simulink model "Simulador_MotorDC_Equivalent_BLDC"  (R2019a)
settings: Solver=VariableStepAuto  StartTime=0.0  StopTime=100  RelTol=1e-3
values from neighbouring files (symbols this model uses):
  b = 3.2*10^(-3)    (= 0.0032)    [Simulador_MotorDC_Equivalent_BLDC.m]
  B_fault = 0    [Simulador_MotorDC_Equivalent_BLDC.m]
  B_nonlinear = 1    [Simulador_MotorDC_Equivalent_BLDC.m]
  delta_load = 0.05    [Simulador_MotorDC_Equivalent_BLDC.m]
  f_i = 0    [Simulador_MotorDC_Equivalent_BLDC.m]
  J = 50*10^(-3)*10^(-4)    (= 5e-06)    [Simulador_MotorDC_Equivalent_BLDC.m]
  J_fault = 0    [Simulador_MotorDC_Equivalent_BLDC.m]
  J_nonlinear = 1    [Simulador_MotorDC_Equivalent_BLDC.m]
  Ke = 0.0745    [Simulador_MotorDC_Equivalent_BLDC.m]
  Kt = 74.5*10^(-3)    (= 0.0745)    [Simulador_MotorDC_Equivalent_BLDC.m]
  L = length(r1)    [Algorisme_FDI.m]    (also in Simulador_MotorDC_Equivalent_BLDC.m = 0.0076)
  L_fault = 0    [Simulador_MotorDC_Equivalent_BLDC.m]
  L_nonlinear = 1    [Simulador_MotorDC_Equivalent_BLDC.m]
  Load_fault = 2*delta_load    (= 0.1)    [Simulador_MotorDC_Equivalent_BLDC.m]
  noise_amp = 0.07    [Simulador_MotorDC_Equivalent_BLDC.m]
  P_V_encoder = 1024    [Simulador_MotorDC_Equivalent_BLDC.m]
  pos_stuck = 0    [Simulador_MotorDC_Equivalent_BLDC.m]
  R = 2*1.72    (= 3.44)    [Simulador_MotorDC_Equivalent_BLDC.m]
  R_fault = 0    [Simulador_MotorDC_Equivalent_BLDC.m]
  R_nonlinear = 1    [Simulador_MotorDC_Equivalent_BLDC.m]
  ramp_f_B = 0    [Simulador_MotorDC_Equivalent_BLDC.m]
  ramp_f_J = 0    [Simulador_MotorDC_Equivalent_BLDC.m]
  ramp_f_L = 0    [Simulador_MotorDC_Equivalent_BLDC.m]
  ramp_f_Load = abrup_incip    (= 1)    [Simulador_MotorDC_Equivalent_BLDC.m]
  ramp_f_R = 0    [Simulador_MotorDC_Equivalent_BLDC.m]
  ramp_f_Vdc = 0    [Simulador_MotorDC_Equivalent_BLDC.m]
  ramp_i = 0    [Simulador_MotorDC_Equivalent_BLDC.m]
  stuck_duration = 1    [Simulador_MotorDC_Equivalent_BLDC.m]
  t_fault = 10    [Simulador_MotorDC_Equivalent_BLDC.m]
  tol_B = 0.05    [Simulador_MotorDC_Equivalent_BLDC.m]
  tol_J = 0.05    [Simulador_MotorDC_Equivalent_BLDC.m]
  tol_L = 0.05    [Simulador_MotorDC_Equivalent_BLDC.m]
  tol_R = 0.01    [Simulador_MotorDC_Equivalent_BLDC.m]
  Tsc = 0.0001    [Simulador_MotorDC_Equivalent_BLDC.m]
  Tsd = 0.0001    [Algorisme_FDI.m]    (also in Simulador_MotorDC_Equivalent_BLDC.m)
  Vdc_fault = 0    [Simulador_MotorDC_Equivalent_BLDC.m]
  vel_B = 0.001    [Simulador_MotorDC_Equivalent_BLDC.m]
  vel_i = 0    [Simulador_MotorDC_Equivalent_BLDC.m]
  vel_J = 0.5    [Simulador_MotorDC_Equivalent_BLDC.m]
  vel_L = 0.1    [Simulador_MotorDC_Equivalent_BLDC.m]
  vel_Load = 0.1    [Simulador_MotorDC_Equivalent_BLDC.m]
  vel_R = 0.001    [Simulador_MotorDC_Equivalent_BLDC.m]
  vel_Vdc = 0.001    [Simulador_MotorDC_Equivalent_BLDC.m]
libraries: simulink x2
settings Model: Creator=quimb  LastModifiedBy=Usuario

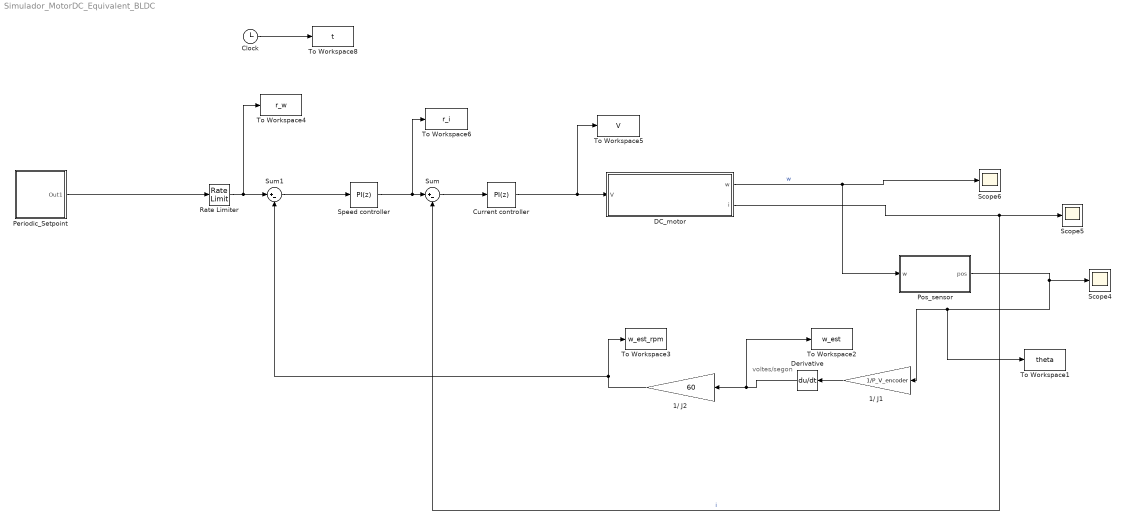
== system Simulador_MotorDC_Equivalent_BLDC ==
  note: voltes/segon
  1/ J1 : Gain  Gain=1/P_V_encoder
  1/ J2 : Gain  Gain=60
  Clock : Clock
  Current controller : simulink/Continuous/PID Controller  Controller=PI  Form=Parallel  TimeDomain=Discrete-time  SampleTime=Tsc  IntegratorMethod=Forward Euler  FilterMethod=Forward Euler  ControllerParametersSource=internal  P=0.1  I=0.1  D=0.5  UseFilter=on  N=100  TunerSelectOption=Transfer Function Based (PID Tuner App)  InitialConditionSource=internal  InitialConditionForIntegrator=0  InitialConditionForFilter=0  DifferentiatorICPrevScaledInput=0  ExternalReset=none  TrackingMode=off  Kt=1  LimitOutput=on  UpperSaturationLimit=24  LowerSaturationLimit=-24  LinearizeAsGain=on  AntiWindupMode=back-calculation  Kb=100  POutMin=[]  POutMax=[]  IOutMin=[]  IOutMax=[]  DOutMin=[]  DOutMax=[]  NOutMin=[]  NOutMax=[]  SumOutMin=[]  SumOutMax=[]  SaturationOutMin=[]  SaturationOutMax=[]  PParamMin=[]  PParamMax=[]  IParamMin=[]  IParamMax=[]  DParamMin=[]  DParamMax=[]  NParamMin=[]  NParamMax=[]  KbParamMin=[]  KbParamMax=[]  KtParamMin=[]  KtParamMax=[]  KbOutMin=[]  KbOutMax=[]  KtOutMin=[]  KtOutMax=[]  IntegratorOutMin=[]  IntegratorOutMax=[]  FilterOutMin=[]  FilterOutMax=[]  SumI1OutMin=[]  SumI1OutMax=[]  SumI2OutMin=[]  SumI2OutMax=[]  SumI3OutMin=[]  SumI3OutMax=[]  SumI4OutMin=[]  SumI4OutMax=[]  SumDOutMin=[]  SumDOutMax=[]  DifferentiatorOutMin=[]  DifferentiatorOutMax=[]  FilterDiffOutCoefMin=[]  FilterDiffOutCoefMax=[]  ReciprocalOutMin=[]  ReciprocalOutMax=[]  SumDenOutMin=[]  SumDenOutMax=[]  SumNumOutMin=[]  SumNumOutMax=[]  DivideOutMin=[]  DivideOutMax=[]  IntegratorContinuousStateAttributes=''  IntegratorStateMustResolveToSignalObject=off  IntegratorRTWStateStorageClass=Auto  FilterContinuousStateAttributes=''  FilterStateMustResolveToSignalObject=off  FilterRTWStateStorageClass=Auto  ParallelPVariant=InternalParameters  IdealPVariant=Disabled  IVariant=InternalParameters  DVariant=Disabled  IntegratorVariant=Discrete  SatVariant=Enabled  AWVariant=BackCalculation  PCopyVariant=Disabled  TRVariant=Disabled  FdbkBlocksVariant=Forward  IdealPFdbkVariant=Disabled  SatFdbkVariant=Disabled  DerivativeFilterVariant=Disabled  NVariant=Disabled  NCopyVariant=Disabled_SignalSpec  FilterICVariant=Disabled  IntegratorICVariant=InternalICs  ExternalResetVariant=Disabled  TRSumVariant=Passthrough  SumFdbkVariant=Disabled  SumVariant=Sum_PI
  DC_motor : Subsystem
  Derivative : Derivative
  Periodic_Setpoint : Subsystem
  Pos_sensor : Subsystem
  Rate Limiter : RateLimiter  RisingSlewLimit=500  FallingSlewLimit=-500  SampleTimeMode=inherited
  Scope4 : Scope
  Scope5 : Scope
  Scope6 : Scope
  Speed controller : simulink/Continuous/PID Controller  Controller=PI  Form=Parallel  TimeDomain=Discrete-time  SampleTime=Tsc  IntegratorMethod=Forward Euler  FilterMethod=Forward Euler  ControllerParametersSource=internal  P=0.5  I=2  D=0.5  UseFilter=on  N=100  TunerSelectOption=Transfer Function Based (PID Tuner App)  InitialConditionSource=internal  InitialConditionForIntegrator=0  InitialConditionForFilter=0  DifferentiatorICPrevScaledInput=0  ExternalReset=none  TrackingMode=off  Kt=1  LimitOutput=on  UpperSaturationLimit=100  LowerSaturationLimit=-100  LinearizeAsGain=on  AntiWindupMode=back-calculation  Kb=100  POutMin=[]  POutMax=[]  IOutMin=[]  IOutMax=[]  DOutMin=[]  DOutMax=[]  NOutMin=[]  NOutMax=[]  SumOutMin=[]  SumOutMax=[]  SaturationOutMin=[]  SaturationOutMax=[]  PParamMin=[]  PParamMax=[]  IParamMin=[]  IParamMax=[]  DParamMin=[]  DParamMax=[]  NParamMin=[]  NParamMax=[]  KbParamMin=[]  KbParamMax=[]  KtParamMin=[]  KtParamMax=[]  KbOutMin=[]  KbOutMax=[]  KtOutMin=[]  KtOutMax=[]  IntegratorOutMin=[]  IntegratorOutMax=[]  FilterOutMin=[]  FilterOutMax=[]  SumI1OutMin=[]  SumI1OutMax=[]  SumI2OutMin=[]  SumI2OutMax=[]  SumI3OutMin=[]  SumI3OutMax=[]  SumI4OutMin=[]  SumI4OutMax=[]  SumDOutMin=[]  SumDOutMax=[]  DifferentiatorOutMin=[]  DifferentiatorOutMax=[]  FilterDiffOutCoefMin=[]  FilterDiffOutCoefMax=[]  ReciprocalOutMin=[]  ReciprocalOutMax=[]  SumDenOutMin=[]  SumDenOutMax=[]  SumNumOutMin=[]  SumNumOutMax=[]  DivideOutMin=[]  DivideOutMax=[]  IntegratorContinuousStateAttributes=''  IntegratorStateMustResolveToSignalObject=off  IntegratorRTWStateStorageClass=Auto  FilterContinuousStateAttributes=''  FilterStateMustResolveToSignalObject=off  FilterRTWStateStorageClass=Auto  ParallelPVariant=InternalParameters  IdealPVariant=Disabled  IVariant=InternalParameters  DVariant=Disabled  IntegratorVariant=Discrete  SatVariant=Enabled  AWVariant=BackCalculation  PCopyVariant=Disabled  TRVariant=Disabled  FdbkBlocksVariant=Forward  IdealPFdbkVariant=Disabled  SatFdbkVariant=Disabled  DerivativeFilterVariant=Disabled  NVariant=Disabled  NCopyVariant=Disabled_SignalSpec  FilterICVariant=Disabled  IntegratorICVariant=InternalICs  ExternalResetVariant=Disabled  TRSumVariant=Passthrough  SumFdbkVariant=Disabled  SumVariant=Sum_PI
  Sum : Sum  Inputs=|+-
  Sum1 : Sum  Inputs=|+-
  To Workspace1 : ToWorkspace  VariableName=theta  SampleTime=Tsd
  To Workspace2 : ToWorkspace  VariableName=w_est  SampleTime=Tsd
  To Workspace3 : ToWorkspace  VariableName=w_est_rpm  SampleTime=Tsd
  To Workspace4 : ToWorkspace  VariableName=r_w  SampleTime=Tsd
  To Workspace5 : ToWorkspace  VariableName=V  SampleTime=Tsd
  To Workspace6 : ToWorkspace  VariableName=r_i  SampleTime=Tsd
  To Workspace8 : ToWorkspace  VariableName=t  SampleTime=Tsd
  wires:
  DC_motor/1(w) -> Pos_sensor/1("w "), Scope6/1  "w"
  Clock/1 -> To Workspace8/1
  1/ J1/1 -> Derivative/1
  Pos_sensor/1(pos) -> To Workspace1/1, 1/ J1/1, Scope4/1
  Derivative/1 -> To Workspace2/1, 1/ J2/1
  1/ J2/1 -> Sum1/2, To Workspace3/1
  DC_motor/2(i) -> Scope5/1, Sum/2  "i"
  Current controller/1 -> To Workspace5/1, DC_motor/1(V)
  Sum1/1 -> Speed controller/1
  Periodic_Setpoint/1(Out1) -> Rate Limiter/1
  Rate Limiter/1 -> To Workspace4/1, Sum1/1
  Speed controller/1 -> To Workspace6/1, Sum/1
  Sum/1 -> Current controller/1

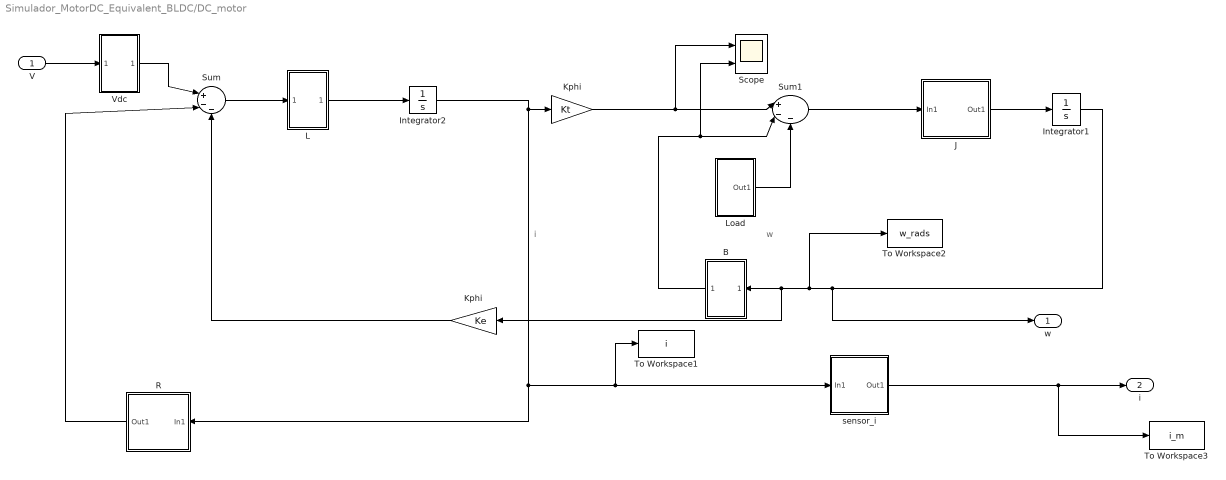
== system Simulador_MotorDC_Equivalent_BLDC/DC_motor ==
  note: i
  note: w
  V : Inport
  B : Subsystem  Tag=R
  Integrator1 : Integrator
  Integrator2 : Integrator
  J : Subsystem
  Kphi : Gain  Gain=Kt
  "Kphi " : Gain  Gain=Ke
  L : Subsystem
  Load : Subsystem
  R : Subsystem  Tag=R
  Scope : Scope  NumInputPorts=2
  Sum : Sum  Inputs=|+--
  Sum1 : Sum  Inputs=|+--
  To Workspace1 : ToWorkspace  VariableName=i  SampleTime=Tsd
  To Workspace2 : ToWorkspace  VariableName=w_rads  SampleTime=Tsd
  To Workspace3 : ToWorkspace  VariableName=i_m  SampleTime=Tsd
  Vdc : Subsystem
  sensor_i : Subsystem  Tag=R
  w : Outport
  i : Outport  Port=2
  wires:
  Sum/1 -> L/1(In1)
  Kphi/1 -> Scope/1, Sum1/1
  L/1(Out1) -> Integrator2/1
  Integrator2/1 -> sensor_i/1(In1), To Workspace1/1, R/1(In1), Kphi/1
  "Kphi "/1 -> Sum/3
  J/1(Out1) -> Integrator1/1
  R/1(Out1) -> Sum/2
  Sum1/1 -> J/1(In1)
  Integrator1/1 -> w/1, To Workspace2/1, B/1(In1), "Kphi "/1
  B/1(Out1) -> Scope/2, Sum1/2
  Load/1(Out1) -> Sum1/3
  sensor_i/1(Out1) -> To Workspace3/1, i/1
  V/1 -> Vdc/1(In1)
  Vdc/1(Out1) -> Sum/1

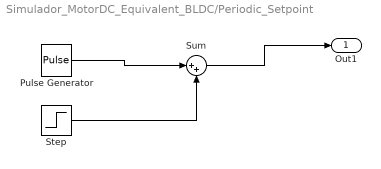
== system Simulador_MotorDC_Equivalent_BLDC/Periodic_Setpoint ==
  Pulse Generator : DiscretePulseGenerator  PulseType=Time based  Amplitude=300  Period=10  PulseWidth=50  PhaseDelay=5
  Step : Step  Before=20  After=20  SampleTime=0
  Sum : Sum  Inputs=|++
  Out1 : Outport
  wires:
  Pulse Generator/1 -> Sum/1
  Step/1 -> Sum/2
  Sum/1 -> Out1/1

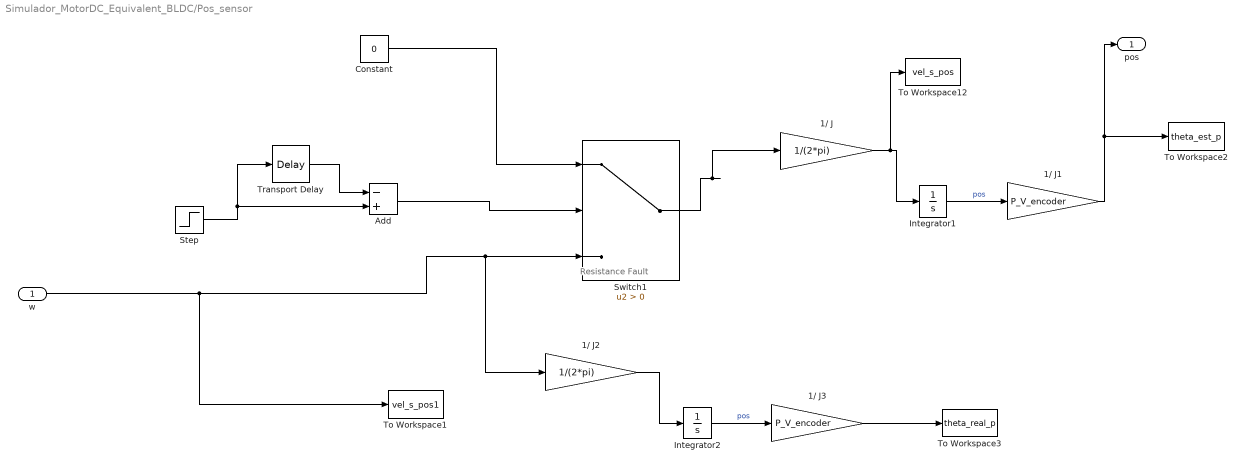
== system Simulador_MotorDC_Equivalent_BLDC/Pos_sensor ==
  note: Resistance Fault
  "w " : Inport
  1/ J : Gain  Gain=1/(2*pi)
  1/ J1 : Gain  Gain=P_V_encoder
  1/ J2 : Gain  Gain=1/(2*pi)
  1/ J3 : Gain  Gain=P_V_encoder
  Add : Sum  Inputs=-+
  Constant : Constant  Value=0
  Integrator1 : Integrator
  Integrator2 : Integrator
  Step : Step  Tag=Rpm Sensor Flow  Time=t_fault  After=pos_stuck  SampleTime=Tsc
  Switch1 : Switch  Criteria=u2 > Threshold
  To Workspace1 : ToWorkspace  VariableName=vel_s_pos1  SampleTime=Tsd
  To Workspace12 : ToWorkspace  VariableName=vel_s_pos  SampleTime=Tsd
  To Workspace2 : ToWorkspace  VariableName=theta_est_p  SampleTime=Tsd
  To Workspace3 : ToWorkspace  VariableName=theta_real_p  SampleTime=Tsd
  Transport Delay : TransportDelay  DelayTime=stuck_duration
  pos : Outport
  wires:
  Constant/1 -> Switch1/1
  "w "/1 -> To Workspace1/1, 1/ J2/1, Switch1/3
  Step/1 -> Add/2, Transport Delay/1
  Transport Delay/1 -> Add/1
  Add/1 -> Switch1/2
  Integrator1/1 -> 1/ J1/1  "pos"
  1/ J1/1 -> To Workspace2/1, pos/1
  1/ J/1 -> To Workspace12/1, Integrator1/1
  Switch1/1 -> 1/ J/1
  1/ J2/1 -> Integrator2/1
  Integrator2/1 -> 1/ J3/1  "pos"
  1/ J3/1 -> To Workspace3/1

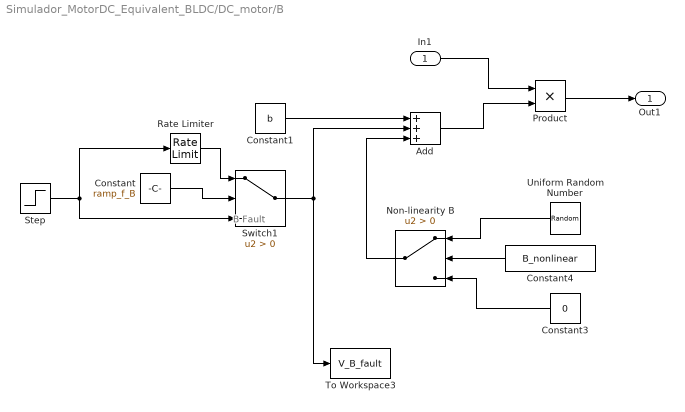
== system Simulador_MotorDC_Equivalent_BLDC/DC_motor/B ==
  note: B Fault
  In1 : Inport
  Add : Sum  Inputs=+++
  Constant : Constant  Value=ramp_f_B
  Constant1 : Constant  Value=b
  Constant3 : Constant  Value=0
  Constant4 : Constant  Value=B_nonlinear
  Non-linearity B : Switch  Criteria=u2 > Threshold
  Product : Product
  Rate Limiter : RateLimiter  RisingSlewLimit=vel_B*b  FallingSlewLimit=-vel_B*b  SampleTimeMode=inherited
  Step : Step  Tag=Rpm Sensor Flow  Time=t_fault  After=B_fault  SampleTime=Tsd
  Switch1 : Switch  Criteria=u2 > Threshold
  To Workspace3 : ToWorkspace  VariableName=V_B_fault  SampleTime=Tsd
  Uniform Random Number : UniformRandomNumber  Minimum=-tol_B*b  Maximum=tol_B*b  SampleTime=Tsd
  Out1 : Outport
  wires:
  Constant/1 -> Switch1/2
  Step/1 -> Switch1/3, Rate Limiter/1
  Rate Limiter/1 -> Switch1/1
  Constant1/1 -> Add/1
  Product/1 -> Out1/1
  Add/1 -> Product/2
  In1/1 -> Product/1
  Constant3/1 -> Non-linearity B/3
  Constant4/1 -> Non-linearity B/2
  Non-linearity B/1 -> Add/3
  Uniform Random Number/1 -> Non-linearity B/1
  Switch1/1 -> To Workspace3/1, Add/2

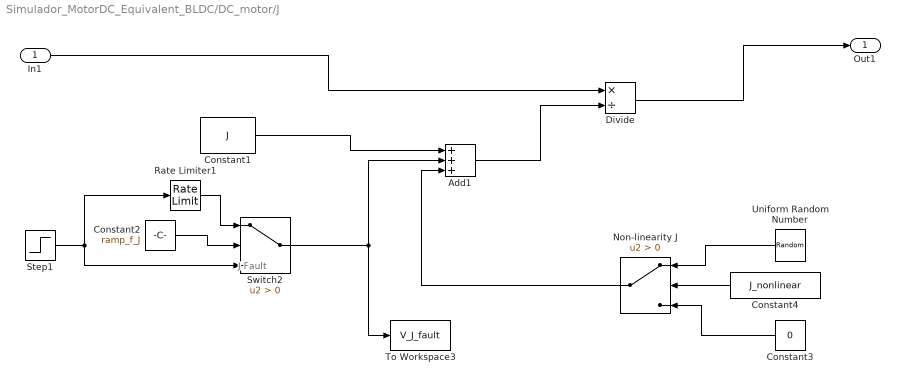
== system Simulador_MotorDC_Equivalent_BLDC/DC_motor/J ==
  note: J Fault
  In1 : Inport
  Add1 : Sum  Inputs=+++
  Constant1 : Constant  Value=J
  Constant2 : Constant  Value=ramp_f_J
  Constant3 : Constant  Value=0
  Constant4 : Constant  Value=J_nonlinear
  Divide : Product  Inputs=*/
  Non-linearity J : Switch  Criteria=u2 > Threshold
  Rate Limiter1 : RateLimiter  RisingSlewLimit=vel_J*J  FallingSlewLimit=-vel_J*J  SampleTimeMode=inherited
  Step1 : Step  Tag=Rpm Sensor Flow  Time=t_fault  After=J_fault  SampleTime=Tsc
  Switch2 : Switch  Criteria=u2 > Threshold
  To Workspace3 : ToWorkspace  VariableName=V_J_fault  SampleTime=Tsd
  Uniform Random Number : UniformRandomNumber  Minimum=-tol_J*J  Maximum=tol_J*J  SampleTime=Tsd
  Out1 : Outport
  wires:
  Rate Limiter1/1 -> Switch2/1
  Step1/1 -> Rate Limiter1/1, Switch2/3
  Constant2/1 -> Switch2/2
  Add1/1 -> Divide/2
  Divide/1 -> Out1/1
  In1/1 -> Divide/1
  Constant1/1 -> Add1/1
  Constant3/1 -> Non-linearity J/3
  Constant4/1 -> Non-linearity J/2
  Non-linearity J/1 -> Add1/3
  Uniform Random Number/1 -> Non-linearity J/1
  Switch2/1 -> To Workspace3/1, Add1/2

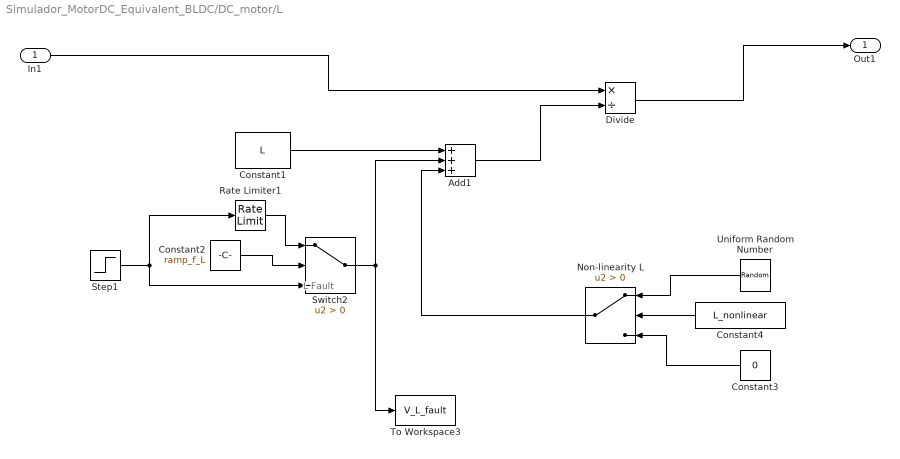
== system Simulador_MotorDC_Equivalent_BLDC/DC_motor/L ==
  note: L Fault
  In1 : Inport
  Add1 : Sum  Inputs=+++
  Constant1 : Constant  Value=L
  Constant2 : Constant  Value=ramp_f_L
  Constant3 : Constant  Value=0
  Constant4 : Constant  Value=L_nonlinear
  Divide : Product  Inputs=*/
  Non-linearity L : Switch  Criteria=u2 > Threshold
  Rate Limiter1 : RateLimiter  RisingSlewLimit=vel_L*L  FallingSlewLimit=-vel_L*L  SampleTimeMode=inherited
  Step1 : Step  Tag=Rpm Sensor Flow  Time=t_fault  After=L_fault  SampleTime=Tsc
  Switch2 : Switch  Criteria=u2 > Threshold
  To Workspace3 : ToWorkspace  VariableName=V_L_fault  SampleTime=Tsd
  Uniform Random Number : UniformRandomNumber  Minimum=-tol_L*L  Maximum=tol_L*L  SampleTime=Tsd
  Out1 : Outport
  wires:
  Constant1/1 -> Add1/1
  In1/1 -> Divide/1
  Divide/1 -> Out1/1
  Add1/1 -> Divide/2
  Constant2/1 -> Switch2/2
  Step1/1 -> Switch2/3, Rate Limiter1/1
  Rate Limiter1/1 -> Switch2/1
  Uniform Random Number/1 -> Non-linearity L/1
  Constant4/1 -> Non-linearity L/2
  Constant3/1 -> Non-linearity L/3
  Non-linearity L/1 -> Add1/3
  Switch2/1 -> To Workspace3/1, Add1/2

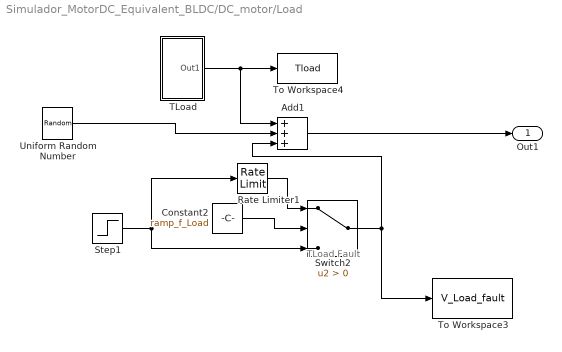
== system Simulador_MotorDC_Equivalent_BLDC/DC_motor/Load ==
  note: TLoad Fault
  Add1 : Sum  Inputs=+++
  Constant2 : Constant  Value=ramp_f_Load
  Rate Limiter1 : RateLimiter  RisingSlewLimit=vel_Load*Load_fault  FallingSlewLimit=-vel_Load*Load_fault  SampleTimeMode=inherited
  Step1 : Step  Tag=Rpm Sensor Flow  Time=t_fault  After=Load_fault  SampleTime=Tsd
  Switch2 : Switch  Criteria=u2 > Threshold
  TLoad : Subsystem
  To Workspace3 : ToWorkspace  VariableName=V_Load_fault  SampleTime=Tsd
  To Workspace4 : ToWorkspace  VariableName=Tload  SampleTime=Tsd
  Uniform Random Number : UniformRandomNumber  Minimum=-delta_load  Maximum=delta_load  SampleTime=Tsd
  Out1 : Outport
  wires:
  Rate Limiter1/1 -> Switch2/1
  Switch2/1 -> Add1/3, To Workspace3/1
  Step1/1 -> Rate Limiter1/1, Switch2/3
  Constant2/1 -> Switch2/2
  Add1/1 -> Out1/1
  Uniform Random Number/1 -> Add1/2
  TLoad/1(Out1) -> To Workspace4/1, Add1/1

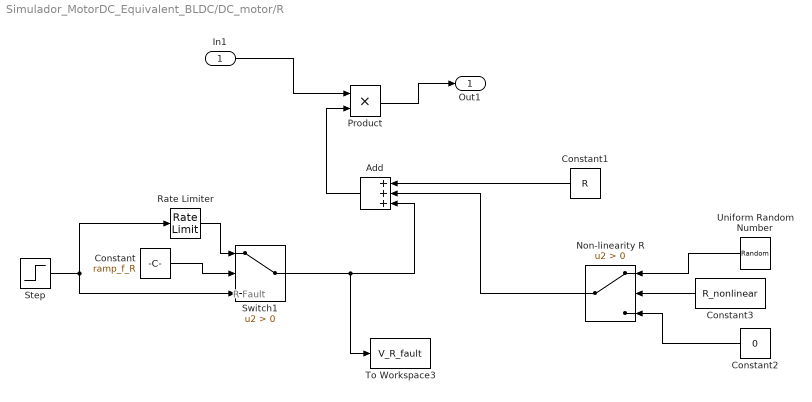
== system Simulador_MotorDC_Equivalent_BLDC/DC_motor/R ==
  note: R Fault
  In1 : Inport
  Add : Sum  Inputs=+++
  Constant : Constant  Value=ramp_f_R
  Constant1 : Constant  Value=R
  Constant2 : Constant  Value=0
  Constant3 : Constant  Value=R_nonlinear
  Non-linearity R : Switch  Criteria=u2 > Threshold
  Product : Product
  Rate Limiter : RateLimiter  RisingSlewLimit=vel_R  FallingSlewLimit=-vel_R  SampleTimeMode=inherited
  Step : Step  Tag=Rpm Sensor Flow  Time=t_fault  After=R_fault  SampleTime=Tsc
  Switch1 : Switch  Criteria=u2 > Threshold
  To Workspace3 : ToWorkspace  VariableName=V_R_fault  SampleTime=Tsd
  Uniform Random Number : UniformRandomNumber  Minimum=-tol_R*R  Maximum=tol_R*R  SampleTime=Tsd
  Out1 : Outport
  wires:
  Rate Limiter/1 -> Switch1/1
  Step/1 -> Rate Limiter/1, Switch1/3
  Constant/1 -> Switch1/2
  Constant1/1 -> Add/1
  In1/1 -> Product/1
  Add/1 -> Product/2
  Product/1 -> Out1/1
  Uniform Random Number/1 -> Non-linearity R/1
  Constant2/1 -> Non-linearity R/3
  Constant3/1 -> Non-linearity R/2
  Non-linearity R/1 -> Add/2
  Switch1/1 -> To Workspace3/1, Add/3

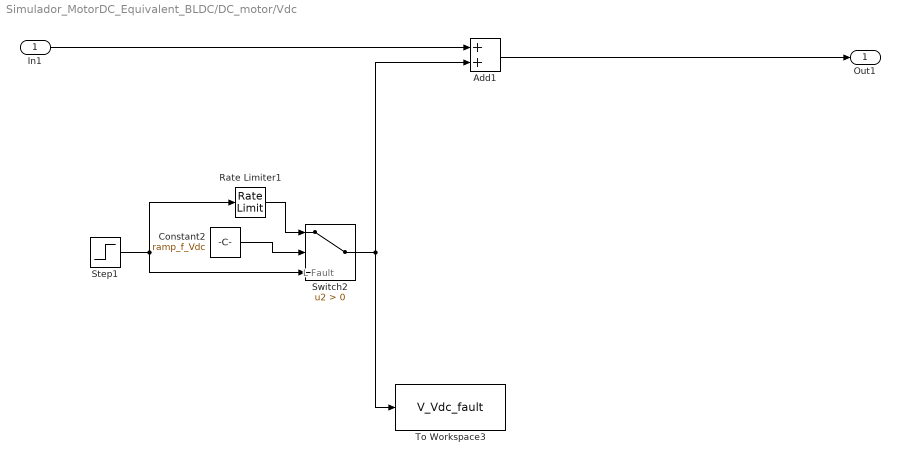
== system Simulador_MotorDC_Equivalent_BLDC/DC_motor/Vdc ==
  note: L Fault
  In1 : Inport
  Add1 : Sum
  Constant2 : Constant  Value=ramp_f_Vdc
  Rate Limiter1 : RateLimiter  RisingSlewLimit=vel_Vdc  FallingSlewLimit=-vel_Vdc  SampleTimeMode=inherited
  Step1 : Step  Tag=Rpm Sensor Flow  Time=t_fault  After=Vdc_fault  SampleTime=Tsc
  Switch2 : Switch  Criteria=u2 > Threshold
  To Workspace3 : ToWorkspace  VariableName=V_Vdc_fault  SampleTime=Tsd
  Out1 : Outport
  wires:
  Switch2/1 -> Add1/2, To Workspace3/1
  Rate Limiter1/1 -> Switch2/1
  Step1/1 -> Rate Limiter1/1, Switch2/3
  Constant2/1 -> Switch2/2
  In1/1 -> Add1/1
  Add1/1 -> Out1/1

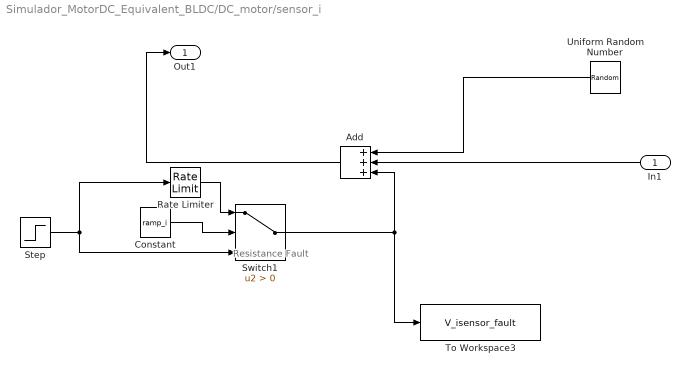
== system Simulador_MotorDC_Equivalent_BLDC/DC_motor/sensor_i ==
  note: Resistance Fault
  In1 : Inport
  Add : Sum  Inputs=+++
  Constant : Constant  Value=ramp_i
  Rate Limiter : RateLimiter  RisingSlewLimit=vel_i  FallingSlewLimit=-vel_i  SampleTimeMode=inherited
  Step : Step  Tag=Rpm Sensor Flow  Time=t_fault  After=f_i  SampleTime=Tsc
  Switch1 : Switch  Criteria=u2 > Threshold
  To Workspace3 : ToWorkspace  VariableName=V_isensor_fault  SampleTime=Tsd
  Uniform Random Number : UniformRandomNumber  Minimum=-noise_amp  Maximum=noise_amp  SampleTime=Tsd
  Out1 : Outport
  wires:
  Rate Limiter/1 -> Switch1/1
  Switch1/1 -> Add/3, To Workspace3/1
  Step/1 -> Rate Limiter/1, Switch1/3
  Constant/1 -> Switch1/2
  Add/1 -> Out1/1
  Uniform Random Number/1 -> Add/1
  In1/1 -> Add/2

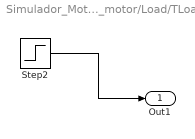
== system Simulador_MotorDC_Equivalent_BLDC/DC_motor/Load/TLoad ==
  Step2 : Step  Tag=Rpm Sensor Flow  After=0  SampleTime=Tsd
  Out1 : Outport
  wires:
  Step2/1 -> Out1/1
